simulink model "Fuzzy_sim_new2"  (R2022a)
settings: Solver=VariableStepAuto  StartTime=0.0  StopTime=100  RelTol=1e-3
values from neighbouring files (symbols this model uses):
  freq_w = 2*pi*freq_hz    (= 2.51327412287)    [Fuzzy_pid.m]
  radius = 0.05    [Fuzzy_pid.m]
  sat_lb = -(pi/180)*5    (= -0.0872664625997)    [Fuzzy_pid.m]
  sat_ub = (pi/180)*5    (= 0.0872664625997)    [Fuzzy_pid.m]
libraries: slpidlib x2, fuzblock x2
settings Model: Creator=Nyz  LastModifiedBy=Nyz
settings ModelReferenceCC: EnableRefExpFcnMdlSchedulingChecks=off
settings RTWCC: Description=Generic Real-Time Target

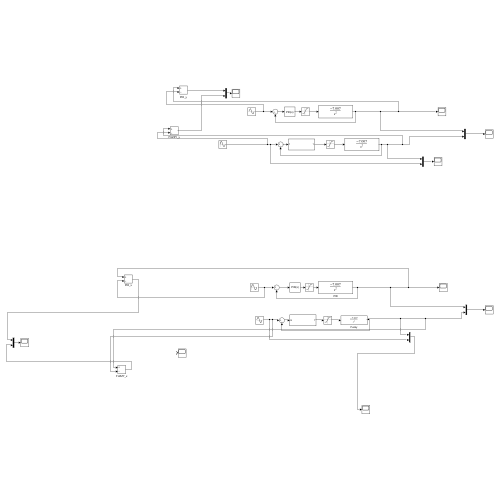
[thumbnail: Simulink's stored preview of the top-level diagram]
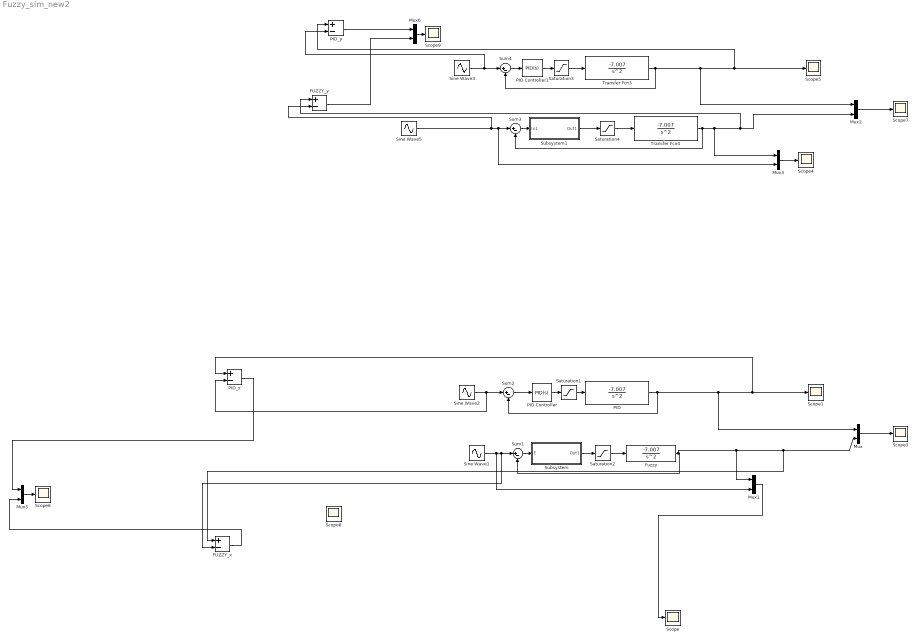
== system Fuzzy_sim_new2 ==
  FUZZY_x : Sum  Inputs=+-
  FUZZY_y : Sum  Inputs=+-
  Fuzzy : TransferFcn  Numerator=[-7.007]  Denominator=[1 0 0]
  Mux{,1..3,5..6} (6 alike) : Mux  Inputs=2
  PID : TransferFcn  Numerator=[-7.007]  Denominator=[1 0 0]
  PID Controller : slpidlib/PID Controller  Controller=PID  Form=Parallel  TimeDomain=Continuous-time  UseExternalTs=off  SampleTime=-1  IntegratorMethod=Forward Euler  FilterMethod=Forward Euler  ControllerParametersSource=internal  P=-15.248335277286007  I=-17.124007265757687  UseKiTs=off  D=-3.334131697914507  N=100  UseFilter=on  TunerSelectOption=Transfer Function Based (PID Tuner App)  InitialConditionSource=internal  InitialConditionForIntegrator=0  InitialConditionForFilter=0  DifferentiatorICPrevScaledInput=0  ExternalReset=none  TrackingMode=off  Kt=1  LimitOutput=off  SatLimitsSource=internal  UpperSaturationLimit=inf  LowerSaturationLimit=-inf  LinearizeAsGain=on  AntiWindupMode=none  Kb=1  POutMin=[]  POutMax=[]  IOutMin=[]  IOutMax=[]  DOutMin=[]  DOutMax=[]  NOutMin=[]  NOutMax=[]  SumOutMin=[]  SumOutMax=[]  SaturationOutMin=[]  SaturationOutMax=[]  PParamMin=[]  PParamMax=[]  IParamMin=[]  IParamMax=[]  DParamMin=[]  DParamMax=[]  NParamMin=[]  NParamMax=[]  KbParamMin=[]  KbParamMax=[]  KtParamMin=[]  KtParamMax=[]  KbOutMin=[]  KbOutMax=[]  KtOutMin=[]  KtOutMax=[]  IntegratorOutMin=[]  IntegratorOutMax=[]  FilterOutMin=[]  FilterOutMax=[]  SumI1OutMin=[]  SumI1OutMax=[]  SumI2OutMin=[]  SumI2OutMax=[]  SumI3OutMin=[]  SumI3OutMax=[]  SumI4OutMin=[]  SumI4OutMax=[]  SumDOutMin=[]  SumDOutMax=[]  DifferentiatorOutMin=[]  DifferentiatorOutMax=[]  FilterDiffOutCoefMin=[]  FilterDiffOutCoefMax=[]  ReciprocalOutMin=[]  ReciprocalOutMax=[]  SumDenOutMin=[]  SumDenOutMax=[]  SumNumOutMin=[]  SumNumOutMax=[]  DivideOutMin=[]  DivideOutMax=[]  UdiffTsProdOutMin=[]  UdiffTsProdOutMax=[]  NTsProdOutMin=[]  NTsProdOutMax=[]  UintegralTsProdOutMin=[]  UintegralTsProdOutMax=[]  UngainTsProdOutMin=[]  UngainTsProdOutMax=[]  IntegratorContinuousStateAttributes=''  IntegratorStateMustResolveToSignalObject=off  IntegratorRTWStateStorageClass=Auto  FilterContinuousStateAttributes=''  FilterStateMustResolveToSignalObject=off  FilterRTWStateStorageClass=Auto  ParallelPVariant=InternalParameters  IdealPVariant=Disabled  IVariant=InternalParameters  DVariant=InternalParameters  IntegratorVariant=Continuous  SatVariant=Disabled  AWVariant=Passthrough  PCopyVariant=Disabled  TRVariant=Disabled  FdbkBlocksVariant=Forward  IdealPFdbkVariant=Disabled  SatFdbkVariant=Disabled  DerivativeFilterVariant=ContFilter  NVariant=InternalParameters  NCopyVariant=Disabled  FilterICVariant=InternalICsFilter  IntegratorICVariant=InternalICs  ExternalResetVariant=Disabled  TRSumVariant=Passthrough  SumFdbkVariant=Disabled  SumVariant=Sum_PID  TsampFilterVariant=InternalTs  TsampNgainVariant=Passthrough  TsampIntegralVariant=Passthrough  ExternalSaturationOutDataTypeStr=Inherit: Same as second input
  PID Controller1 : slpidlib/PID Controller  Controller=PID  Form=Parallel  TimeDomain=Continuous-time  UseExternalTs=off  SampleTime=-1  IntegratorMethod=Forward Euler  FilterMethod=Forward Euler  ControllerParametersSource=internal  P=-15.248335277286007  I=-17.124007265757687  UseKiTs=off  D=-3.334131697914507  N=100  UseFilter=on  TunerSelectOption=Transfer Function Based (PID Tuner App)  InitialConditionSource=internal  InitialConditionForIntegrator=0  InitialConditionForFilter=0  DifferentiatorICPrevScaledInput=0  ExternalReset=none  TrackingMode=off  Kt=1  LimitOutput=off  SatLimitsSource=internal  UpperSaturationLimit=inf  LowerSaturationLimit=-inf  LinearizeAsGain=on  AntiWindupMode=none  Kb=1  POutMin=[]  POutMax=[]  IOutMin=[]  IOutMax=[]  DOutMin=[]  DOutMax=[]  NOutMin=[]  NOutMax=[]  SumOutMin=[]  SumOutMax=[]  SaturationOutMin=[]  SaturationOutMax=[]  PParamMin=[]  PParamMax=[]  IParamMin=[]  IParamMax=[]  DParamMin=[]  DParamMax=[]  NParamMin=[]  NParamMax=[]  KbParamMin=[]  KbParamMax=[]  KtParamMin=[]  KtParamMax=[]  KbOutMin=[]  KbOutMax=[]  KtOutMin=[]  KtOutMax=[]  IntegratorOutMin=[]  IntegratorOutMax=[]  FilterOutMin=[]  FilterOutMax=[]  SumI1OutMin=[]  SumI1OutMax=[]  SumI2OutMin=[]  SumI2OutMax=[]  SumI3OutMin=[]  SumI3OutMax=[]  SumI4OutMin=[]  SumI4OutMax=[]  SumDOutMin=[]  SumDOutMax=[]  DifferentiatorOutMin=[]  DifferentiatorOutMax=[]  FilterDiffOutCoefMin=[]  FilterDiffOutCoefMax=[]  ReciprocalOutMin=[]  ReciprocalOutMax=[]  SumDenOutMin=[]  SumDenOutMax=[]  SumNumOutMin=[]  SumNumOutMax=[]  DivideOutMin=[]  DivideOutMax=[]  UdiffTsProdOutMin=[]  UdiffTsProdOutMax=[]  NTsProdOutMin=[]  NTsProdOutMax=[]  UintegralTsProdOutMin=[]  UintegralTsProdOutMax=[]  UngainTsProdOutMin=[]  UngainTsProdOutMax=[]  IntegratorContinuousStateAttributes=''  IntegratorStateMustResolveToSignalObject=off  IntegratorRTWStateStorageClass=Auto  FilterContinuousStateAttributes=''  FilterStateMustResolveToSignalObject=off  FilterRTWStateStorageClass=Auto  ParallelPVariant=InternalParameters  IdealPVariant=Disabled  IVariant=InternalParameters  DVariant=InternalParameters  IntegratorVariant=Continuous  SatVariant=Disabled  AWVariant=Passthrough  PCopyVariant=Disabled  TRVariant=Disabled  FdbkBlocksVariant=Forward  IdealPFdbkVariant=Disabled  SatFdbkVariant=Disabled  DerivativeFilterVariant=ContFilter  NVariant=InternalParameters  NCopyVariant=Disabled  FilterICVariant=InternalICsFilter  IntegratorICVariant=InternalICs  ExternalResetVariant=Disabled  TRSumVariant=Passthrough  SumFdbkVariant=Disabled  SumVariant=Sum_PID  TsampFilterVariant=InternalTs  TsampNgainVariant=Passthrough  TsampIntegralVariant=Passthrough  ExternalSaturationOutDataTypeStr=Inherit: Same as second input
  PID_x : Sum  Inputs=+-
  PID_y : Sum  Inputs=+-
  Saturation{1..4} (4 alike) : Saturate  UpperLimit=sat_ub  LowerLimit=sat_lb
  Scope{,1,3..9} (9 alike) : Scope
  Sine Wave1 : Sin  Amplitude=radius  Frequency=freq_w  Phase=pi/2  SampleTime=0
  Sine Wave2 : Sin  Amplitude=radius  Frequency=freq_w  Phase=pi/2  SampleTime=0
  Sine Wave3 : Sin  Amplitude=radius  Frequency=freq_w  SampleTime=0
  Sine Wave5 : Sin  Amplitude=radius  Frequency=freq_w  SampleTime=0
  Subsystem : Subsystem
  Subsystem1 : Subsystem
  Sum{1..4} (4 alike) : Sum  Inputs=|+-  InputSameDT=on  SaturateOnIntegerOverflow=on  OutDataTypeStr=Inherit: Same as first input
  Transfer Fcn3 : TransferFcn  Numerator=[-7.007]  Denominator=[1 0 0]
  Transfer Fcn4 : TransferFcn  Numerator=[-7.007]  Denominator=[1 0 0]
  wires:
  PID/1 -> Sum2/2, Mux/1, PID_x/1, Scope1/1
  Sine Wave2/1 -> PID_x/2, Sum2/1
  Sum2/1 -> PID Controller/1
  Sine Wave1/1 -> FUZZY_x/2, Sum1/1, Mux1/2
  Sum1/1 -> Subsystem/1(E)
  Mux/1 -> Scope3/1
  Mux1/1 -> Scope/1
  Fuzzy/1 -> FUZZY_x/1, Mux/2, Mux1/1, Sum1/2
  Mux2/1 -> Scope7/1
  Mux3/1 -> Scope4/1
  Sum4/1 -> PID Controller1/1
  Transfer Fcn4/1 -> Sum3/2, FUZZY_y/1, Mux2/2, Mux3/1
  Sum3/1 -> Subsystem1/1(In1)
  Sine Wave3/1 -> PID_y/2, Sum4/1
  Transfer Fcn3/1 -> Sum4/2, Mux2/1, PID_y/1, Scope5/1
  Sine Wave5/1 -> FUZZY_y/2, Mux3/2, Sum3/1
  PID_x/1 -> Mux5/1
  FUZZY_x/1 -> Mux5/2
  Mux5/1 -> Scope6/1
  PID_y/1 -> Mux6/1
  FUZZY_y/1 -> Mux6/2
  Mux6/1 -> Scope9/1
  PID Controller/1 -> Saturation1/1
  PID Controller1/1 -> Saturation3/1
  Subsystem/1(Out1) -> Saturation2/1
  Subsystem1/1(Out1) -> Saturation4/1
  Saturation1/1 -> PID/1
  Saturation2/1 -> Fuzzy/1
  Saturation3/1 -> Transfer Fcn3/1
  Saturation4/1 -> Transfer Fcn4/1

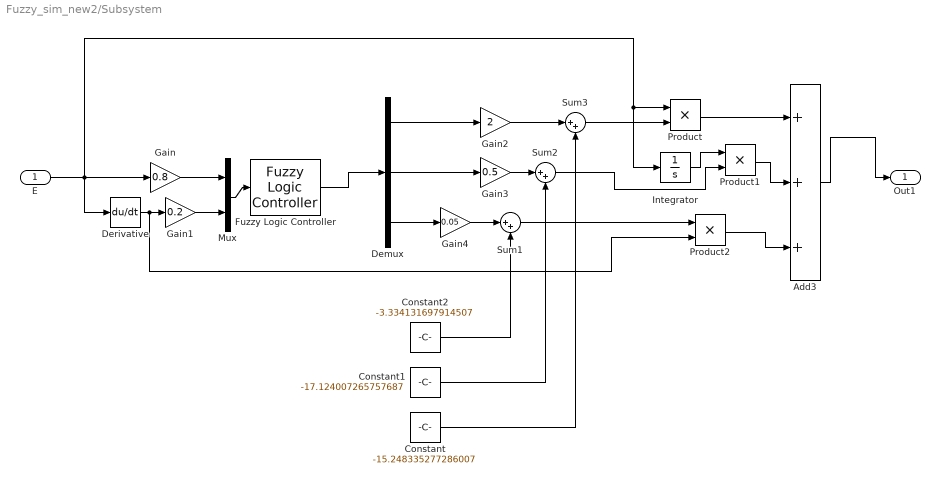
== system Fuzzy_sim_new2/Subsystem ==
  E : Inport
  Add3 : Sum  Inputs=+++
  Constant : Constant  Value=-15.248335277286007
  Constant1 : Constant  Value=-17.124007265757687
  Constant2 : Constant  Value=-3.334131697914507
  Demux : Demux  Outputs=3
  Derivative : Derivative
  Fuzzy Logic Controller : fuzblock/Fuzzy Logic  Controller  FIS='fuzzy2.fis'  OutputSampleNumber=101  DataType=double  FuzzifiedInputs=off  RuleFiringStrengths=off  RuleOutputs=off  AggregatedOutputs=off  SimulateUsing=Interpreted execution  OutOfRangeInputValueMessage=warning  NoRuleFiredMessage=warning  EmptyOutputFuzzySetMessage=warning
  Gain : Gain  Gain=0.8
  Gain1 : Gain  Gain=0.2
  Gain2 : Gain  Gain=2
  Gain3 : Gain  Gain=0.5
  Gain4 : Gain  Gain=0.05
  Integrator : Integrator
  Mux : Mux  Inputs=2
  Product : Product
  Product1 : Product
  Product2 : Product
  Sum1 : Sum  Inputs=|++  InputSameDT=on  SaturateOnIntegerOverflow=on  OutDataTypeStr=Inherit: Same as first input
  Sum2 : Sum  Inputs=|++  InputSameDT=on  SaturateOnIntegerOverflow=on  OutDataTypeStr=Inherit: Same as first input
  Sum3 : Sum  Inputs=|++  InputSameDT=on  SaturateOnIntegerOverflow=on  OutDataTypeStr=Inherit: Same as first input
  Out1 : Outport
  wires:
  Mux/1 -> Fuzzy Logic Controller/1
  E/1 -> Integrator/1, Product/1, Derivative/1, Gain/1
  Derivative/1 -> Product2/2, Gain1/1
  Gain/1 -> Mux/1
  Gain1/1 -> Mux/2
  Fuzzy Logic Controller/1 -> Demux/1
  Demux/1 -> Gain2/1
  Demux/2 -> Gain3/1
  Demux/3 -> Gain4/1
  Sum3/1 -> Product/2
  Product/1 -> Add3/1
  Product1/1 -> Add3/2
  Sum2/1 -> Product1/2
  Integrator/1 -> Product1/1
  Sum1/1 -> Product2/1
  Product2/1 -> Add3/3
  Gain3/1 -> Sum2/1
  Gain4/1 -> Sum1/1
  Add3/1 -> Out1/1
  Constant2/1 -> Sum1/2
  Constant1/1 -> Sum2/2
  Gain2/1 -> Sum3/1
  Constant/1 -> Sum3/2

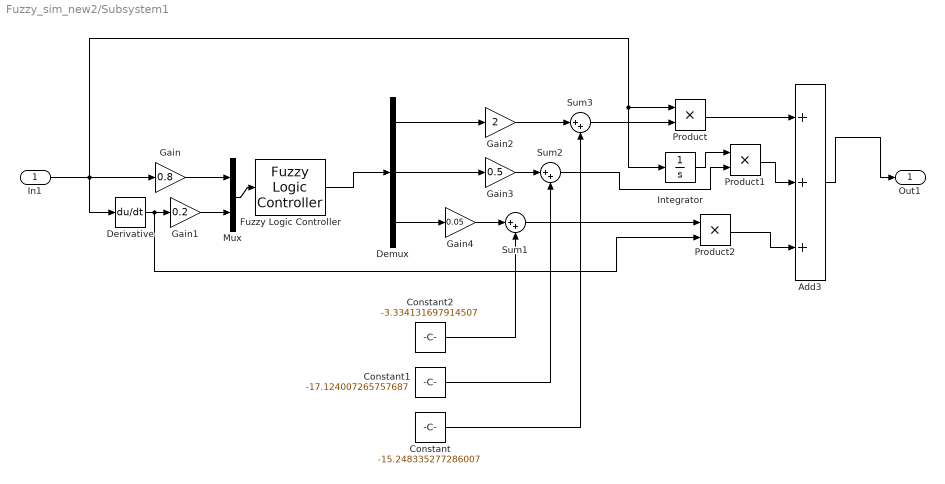
== system Fuzzy_sim_new2/Subsystem1 ==
  In1 : Inport
  Add3 : Sum  Inputs=+++
  Constant : Constant  Value=-15.248335277286007
  Constant1 : Constant  Value=-17.124007265757687
  Constant2 : Constant  Value=-3.334131697914507
  Demux : Demux  Outputs=3
  Derivative : Derivative
  Fuzzy Logic Controller : fuzblock/Fuzzy Logic  Controller  FIS='fuzzy2.fis'  OutputSampleNumber=101  DataType=double  FuzzifiedInputs=off  RuleFiringStrengths=off  RuleOutputs=off  AggregatedOutputs=off  SimulateUsing=Interpreted execution  OutOfRangeInputValueMessage=warning  NoRuleFiredMessage=warning  EmptyOutputFuzzySetMessage=warning
  Gain : Gain  Gain=0.8
  Gain1 : Gain  Gain=0.2
  Gain2 : Gain  Gain=2
  Gain3 : Gain  Gain=0.5
  Gain4 : Gain  Gain=0.05
  Integrator : Integrator
  Mux : Mux  Inputs=2
  Product : Product
  Product1 : Product
  Product2 : Product
  Sum1 : Sum  Inputs=|++  InputSameDT=on  SaturateOnIntegerOverflow=on  OutDataTypeStr=Inherit: Same as first input
  Sum2 : Sum  Inputs=|++  InputSameDT=on  SaturateOnIntegerOverflow=on  OutDataTypeStr=Inherit: Same as first input
  Sum3 : Sum  Inputs=|++  InputSameDT=on  SaturateOnIntegerOverflow=on  OutDataTypeStr=Inherit: Same as first input
  Out1 : Outport
  wires:
  Gain2/1 -> Sum3/1
  Sum3/1 -> Product/2
  Sum2/1 -> Product1/2
  Constant2/1 -> Sum1/2
  Sum1/1 -> Product2/1
  Gain3/1 -> Sum2/1
  Gain4/1 -> Sum1/1
  Constant1/1 -> Sum2/2
  Demux/1 -> Gain2/1
  Product/1 -> Add3/1
  Product2/1 -> Add3/3
  Demux/2 -> Gain3/1
  Fuzzy Logic Controller/1 -> Demux/1
  Gain1/1 -> Mux/2
  Add3/1 -> Out1/1
  Integrator/1 -> Product1/1
  Gain/1 -> Mux/1
  Mux/1 -> Fuzzy Logic Controller/1
  In1/1 -> Integrator/1, Product/1, Derivative/1, Gain/1
  Demux/3 -> Gain4/1
  Constant/1 -> Sum3/2
  Product1/1 -> Add3/2
  Derivative/1 -> Product2/2, Gain1/1
